simulink model "Open_Loop_Control"  (R2023a)
settings: Solver=VariableStepAuto  StartTime=0.0  StopTime=inf  RelTol=1e-3
libraries: instrumentseriallib x2
settings Model: Creator=ela19kfs  LastModifiedBy=ela19kfs

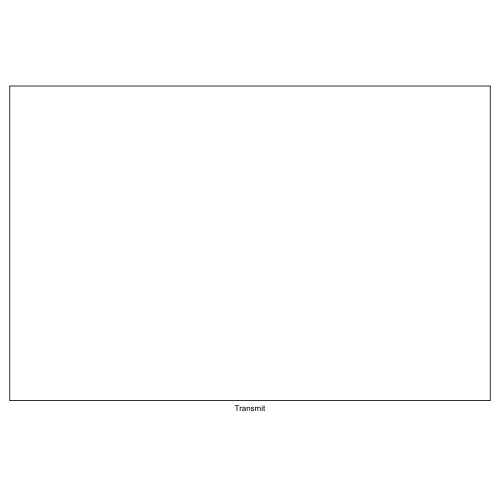
[thumbnail: Simulink's stored preview of the top-level diagram]
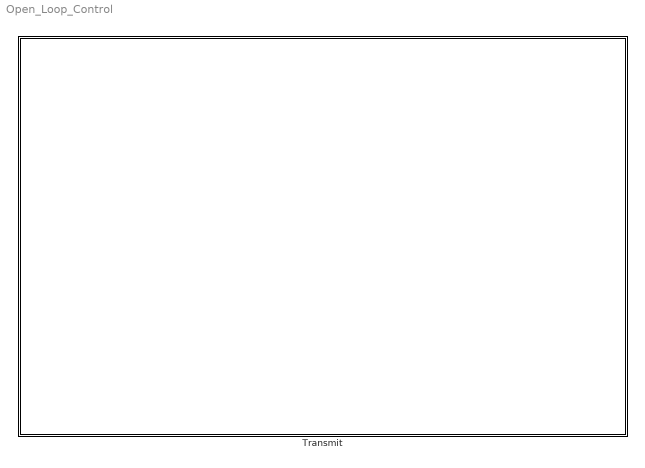
== system Open_Loop_Control ==
  Transmit : Subsystem

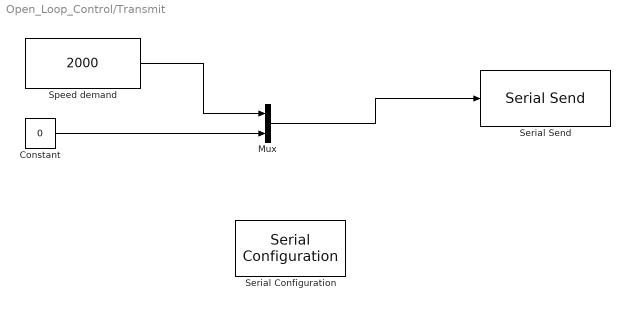
== system Open_Loop_Control/Transmit ==
  Constant : Constant  Value=0  OutDataTypeStr=uint16
  Mux : Mux  Inputs=2
  Serial Configuration : instrumentseriallib/Serial Configuration  Priority=-200000  PortSel=COM7  Port=COM7  ComPort=COM7  BaudRate=5e6  DataBits=8  Parity=none  StopBits=1  ByteOrder=little-endian  FlowControl=none  Timeout=2  SimulateUsing=Interpreted execution  BlockInModel=on  aMode=1
      settings: LibrarySourceBlock=embeddedtargetslib/Host Communication/Serial Configuration
  Serial Send : instrumentseriallib/Serial Send  Priority=1  PortSel=COM7  Port=COM7  ComPort=COM7  Header=[]  Terminator=<none>  CustomTerminator=[]  EnableBlockingMode=on  SimulateUsing=Interpreted execution  BlockInModel=on  aMode=1
  Speed demand : Constant  Value=2000  OutDataTypeStr=uint16
  wires:
  Constant/1 -> Mux/2
  Speed demand/1 -> Mux/1
  Mux/1 -> Serial Send/1
